simulink model "inner_tanks_init"  (R2020a)
settings: Solver=FixedStepAuto  StartTime=0.0  StopTime=inf  FixedStep=1  RelTol=1e-3
libraries: modbusMatLib x12, simulink x4, realtime_pacer_lib x1
(part 1 of 2)
settings Model: Creator=pppc  LastModifiedBy=Casper and Adis
settings DebuggingCC: InheritedTsInSrcMsg=none
settings SFSimCC: CustomCodeUndefinedFunction=UseInterfaceOnly

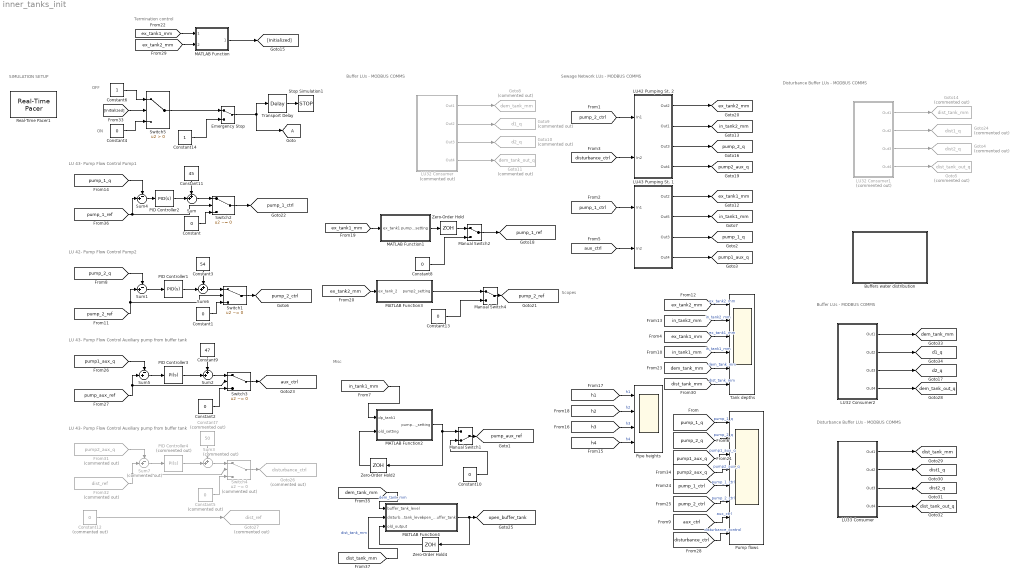
== system inner_tanks_init ==
  note: Buffer LUs - MODBUS COMMS
  note: LU 43- Pump Flow Control Auxiliary pump from buffer tank
  note: OFF
  note: SIMULATION SETUP
  note: Sewage Network LUs - MODBUS COMMS
  note: LU 43- Pump Flow Control Pump1
  note: LU 42- Pump Flow Control Pump2
  note: ON
  note: Scopes
  note: Disturbance Buffer LUs - MODBUS COMMS
  note: LU 43- Pump Flow Control Auxiliary pump from buffer tank
  note: Termination control
  note: Misc
  note: Disturbance Buffer LUs - MODBUS COMMS
  note: Buffer LUs - MODBUS COMMS
  Buffers water distribution : Subsystem
  Constant{,1..2,4,8,10,13} (7 alike) : Constant  Value=0
  Constant11 : Constant  Value=45
  Constant12 : Constant  Commented=on  Value=0
  Constant14 : Constant
  Constant3 : Constant  Value=54
  Constant5 : Constant  Commented=on  Value=0
  Constant6 : Constant
  Constant7 : Constant  Commented=on  Value=50
  Constant9 : Constant  Value=47
  Emergency Stop : ManualSwitch
  From31 : From  Commented=on  GotoTag=pump2_aux_q  TagVisibility=global
  From32 : From  Commented=on  GotoTag=dist_ref  TagVisibility=global
  Goto10 : Goto  Commented=on  GotoTag=d2_q  TagVisibility=global
  Goto11 : Goto  Commented=on  GotoTag=dem_tank_out_q  TagVisibility=global
  Goto14 : Goto  Commented=on  GotoTag=dist_tank_mm  TagVisibility=global
  Goto24 : Goto  Commented=on  GotoTag=dist1_q  TagVisibility=global
  Goto26 : Goto  Commented=on  GotoTag=disturbance_ctrl  TagVisibility=global
  Goto27 : Goto  Commented=on  GotoTag=dist_ref  TagVisibility=global
  Goto4 : Goto  Commented=on  GotoTag=dist2_q  TagVisibility=global
  Goto5 : Goto  Commented=on  GotoTag=dist_tank_out_q  TagVisibility=global
  Goto8 : Goto  Commented=on  GotoTag=dem_tank_mm  TagVisibility=global
  Goto9 : Goto  Commented=on  GotoTag=d1_q  TagVisibility=global
  LU32 Consumer : Subsystem  Commented=on
  LU32 Consumer1 : Subsystem  Commented=on
  LU32 Consumer2 : Subsystem
  LU33 Consumer : Subsystem
  LU42 Pumping St. 2 : Subsystem
  LU43 Pumping St. 1 : Subsystem
  MATLAB Function : MATLAB Function  TreatAsAtomicUnit=on
  MATLAB Function1 : MATLAB Function  TreatAsAtomicUnit=on
  MATLAB Function2 : MATLAB Function  TreatAsAtomicUnit=on
  MATLAB Function3 : MATLAB Function  TreatAsAtomicUnit=on
  MATLAB Function4 : MATLAB Function  TreatAsAtomicUnit=on
  Manual Switch1 : ManualSwitch  CurrentSetting=0
  Manual Switch2 : ManualSwitch
  Manual Switch4 : ManualSwitch
  PID Controller1 : simulink/Continuous/PID Controller  Controller=PID  Form=Parallel  TimeDomain=Continuous-time  UseExternalTs=off  SampleTime=1  IntegratorMethod=Forward Euler  FilterMethod=Forward Euler  ControllerParametersSource=internal  P=0.145  I=0.61  D=0  UseFilter=on  N=100  TunerSelectOption=Transfer Function Based (PID Tuner App)  InitialConditionSource=internal  InitialConditionForIntegrator=0  InitialConditionForFilter=0  DifferentiatorICPrevScaledInput=0  ExternalReset=none  TrackingMode=off  Kt=1  LimitOutput=on  UpperSaturationLimit=46  LowerSaturationLimit=0  LinearizeAsGain=off  AntiWindupMode=clamping  Kb=1  POutMin=[]  POutMax=[]  IOutMin=[]  IOutMax=[]  DOutMin=[]  DOutMax=[]  NOutMin=[]  NOutMax=[]  SumOutMin=[]  SumOutMax=[]  SaturationOutMin=[]  SaturationOutMax=[]  PParamMin=[]  PParamMax=[]  IParamMin=[]  IParamMax=[]  DParamMin=[]  DParamMax=[]  NParamMin=[]  NParamMax=[]  KbParamMin=[]  KbParamMax=[]  KtParamMin=[]  KtParamMax=[]  KbOutMin=[]  KbOutMax=[]  KtOutMin=[]  KtOutMax=[]  IntegratorOutMin=[]  IntegratorOutMax=[]  FilterOutMin=[]  FilterOutMax=[]  SumI1OutMin=[]  SumI1OutMax=[]  SumI2OutMin=[]  SumI2OutMax=[]  SumI3OutMin=[]  SumI3OutMax=[]  SumI4OutMin=[]  SumI4OutMax=[]  SumDOutMin=[]  SumDOutMax=[]  DifferentiatorOutMin=[]  DifferentiatorOutMax=[]  FilterDiffOutCoefMin=[]  FilterDiffOutCoefMax=[]  ReciprocalOutMin=[]  ReciprocalOutMax=[]  SumDenOutMin=[]  SumDenOutMax=[]  SumNumOutMin=[]  SumNumOutMax=[]  DivideOutMin=[]  DivideOutMax=[]  UdiffTsProdOutMin=[]  UdiffTsProdOutMax=[]  NTsProdOutMin=[]  NTsProdOutMax=[]  UintegralTsProdOutMin=[]  UintegralTsProdOutMax=[]  UngainTsProdOutMin=[]  UngainTsProdOutMax=[]  IntegratorContinuousStateAttributes=''  IntegratorStateMustResolveToSignalObject=off  IntegratorRTWStateStorageClass=Auto  FilterContinuousStateAttributes=''  FilterStateMustResolveToSignalObject=off  FilterRTWStateStorageClass=Auto  ParallelPVariant=InternalParameters  IdealPVariant=Disabled  IVariant=InternalParameters  DVariant=InternalParameters  IntegratorVariant=Continuous  SatVariant=Enabled  AWVariant=ContClampingParallel  PCopyVariant=Disabled  TRVariant=Disabled  FdbkBlocksVariant=Forward  IdealPFdbkVariant=Disabled  SatFdbkVariant=Disabled  DerivativeFilterVariant=ContFilter  NVariant=InternalParameters  NCopyVariant=Disabled  FilterICVariant=InternalICsFilter  IntegratorICVariant=InternalICs  ExternalResetVariant=Disabled  TRSumVariant=Passthrough  SumFdbkVariant=Disabled  SumVariant=Sum_PID  TsampFilterVariant=InternalTs  TsampNgainVariant=Passthrough  TsampIntegralVariant=Passthrough
  PID Controller2 : simulink/Continuous/PID Controller  Controller=PID  Form=Parallel  TimeDomain=Continuous-time  UseExternalTs=off  SampleTime=1  IntegratorMethod=Forward Euler  FilterMethod=Forward Euler  ControllerParametersSource=internal  P=0.1  I=0.3  D=0  UseFilter=on  N=100  TunerSelectOption=Transfer Function Based (PID Tuner App)  InitialConditionSource=internal  InitialConditionForIntegrator=0  InitialConditionForFilter=0  DifferentiatorICPrevScaledInput=0  ExternalReset=none  TrackingMode=off  Kt=1  LimitOutput=on  UpperSaturationLimit=49  LowerSaturationLimit=0  LinearizeAsGain=off  AntiWindupMode=clamping  Kb=1  POutMin=[]  POutMax=[]  IOutMin=[]  IOutMax=[]  DOutMin=[]  DOutMax=[]  NOutMin=[]  NOutMax=[]  SumOutMin=[]  SumOutMax=[]  SaturationOutMin=[]  SaturationOutMax=[]  PParamMin=[]  PParamMax=[]  IParamMin=[]  IParamMax=[]  DParamMin=[]  DParamMax=[]  NParamMin=[]  NParamMax=[]  KbParamMin=[]  KbParamMax=[]  KtParamMin=[]  KtParamMax=[]  KbOutMin=[]  KbOutMax=[]  KtOutMin=[]  KtOutMax=[]  IntegratorOutMin=[]  IntegratorOutMax=[]  FilterOutMin=[]  FilterOutMax=[]  SumI1OutMin=[]  SumI1OutMax=[]  SumI2OutMin=[]  SumI2OutMax=[]  SumI3OutMin=[]  SumI3OutMax=[]  SumI4OutMin=[]  SumI4OutMax=[]  SumDOutMin=[]  SumDOutMax=[]  DifferentiatorOutMin=[]  DifferentiatorOutMax=[]  FilterDiffOutCoefMin=[]  FilterDiffOutCoefMax=[]  ReciprocalOutMin=[]  ReciprocalOutMax=[]  SumDenOutMin=[]  SumDenOutMax=[]  SumNumOutMin=[]  SumNumOutMax=[]  DivideOutMin=[]  DivideOutMax=[]  UdiffTsProdOutMin=[]  UdiffTsProdOutMax=[]  NTsProdOutMin=[]  NTsProdOutMax=[]  UintegralTsProdOutMin=[]  UintegralTsProdOutMax=[]  UngainTsProdOutMin=[]  UngainTsProdOutMax=[]  IntegratorContinuousStateAttributes=''  IntegratorStateMustResolveToSignalObject=off  IntegratorRTWStateStorageClass=Auto  FilterContinuousStateAttributes=''  FilterStateMustResolveToSignalObject=off  FilterRTWStateStorageClass=Auto  ParallelPVariant=InternalParameters  IdealPVariant=Disabled  IVariant=InternalParameters  DVariant=InternalParameters  IntegratorVariant=Continuous  SatVariant=Enabled  AWVariant=ContClampingParallel  PCopyVariant=Disabled  TRVariant=Disabled  FdbkBlocksVariant=Forward  IdealPFdbkVariant=Disabled  SatFdbkVariant=Disabled  DerivativeFilterVariant=ContFilter  NVariant=InternalParameters  NCopyVariant=Disabled  FilterICVariant=InternalICsFilter  IntegratorICVariant=InternalICs  ExternalResetVariant=Disabled  TRSumVariant=Passthrough  SumFdbkVariant=Disabled  SumVariant=Sum_PID  TsampFilterVariant=InternalTs  TsampNgainVariant=Passthrough  TsampIntegralVariant=Passthrough
  PID Controller3 : simulink/Continuous/PID Controller  Controller=PI  Form=Parallel  TimeDomain=Continuous-time  UseExternalTs=off  SampleTime=1  IntegratorMethod=Forward Euler  FilterMethod=Forward Euler  ControllerParametersSource=internal  P=0.15  I=0.45  D=0  UseFilter=on  N=100  TunerSelectOption=Transfer Function Based (PID Tuner App)  InitialConditionSource=internal  InitialConditionForIntegrator=0  InitialConditionForFilter=0  DifferentiatorICPrevScaledInput=0  ExternalReset=none  TrackingMode=off  Kt=1  LimitOutput=on  UpperSaturationLimit=53  LowerSaturationLimit=0  LinearizeAsGain=off  AntiWindupMode=clamping  Kb=1  POutMin=[]  POutMax=[]  IOutMin=[]  IOutMax=[]  DOutMin=[]  DOutMax=[]  NOutMin=[]  NOutMax=[]  SumOutMin=[]  SumOutMax=[]  SaturationOutMin=[]  SaturationOutMax=[]  PParamMin=[]  PParamMax=[]  IParamMin=[]  IParamMax=[]  DParamMin=[]  DParamMax=[]  NParamMin=[]  NParamMax=[]  KbParamMin=[]  KbParamMax=[]  KtParamMin=[]  KtParamMax=[]  KbOutMin=[]  KbOutMax=[]  KtOutMin=[]  KtOutMax=[]  IntegratorOutMin=[]  IntegratorOutMax=[]  FilterOutMin=[]  FilterOutMax=[]  SumI1OutMin=[]  SumI1OutMax=[]  SumI2OutMin=[]  SumI2OutMax=[]  SumI3OutMin=[]  SumI3OutMax=[]  SumI4OutMin=[]  SumI4OutMax=[]  SumDOutMin=[]  SumDOutMax=[]  DifferentiatorOutMin=[]  DifferentiatorOutMax=[]  FilterDiffOutCoefMin=[]  FilterDiffOutCoefMax=[]  ReciprocalOutMin=[]  ReciprocalOutMax=[]  SumDenOutMin=[]  SumDenOutMax=[]  SumNumOutMin=[]  SumNumOutMax=[]  DivideOutMin=[]  DivideOutMax=[]  UdiffTsProdOutMin=[]  UdiffTsProdOutMax=[]  NTsProdOutMin=[]  NTsProdOutMax=[]  UintegralTsProdOutMin=[]  UintegralTsProdOutMax=[]  UngainTsProdOutMin=[]  UngainTsProdOutMax=[]  IntegratorContinuousStateAttributes=''  IntegratorStateMustResolveToSignalObject=off  IntegratorRTWStateStorageClass=Auto  FilterContinuousStateAttributes=''  FilterStateMustResolveToSignalObject=off  FilterRTWStateStorageClass=Auto  ParallelPVariant=InternalParameters  IdealPVariant=Disabled  IVariant=InternalParameters  DVariant=Disabled  IntegratorVariant=Continuous  SatVariant=Enabled  AWVariant=ContClampingParallel  PCopyVariant=Disabled  TRVariant=Disabled  FdbkBlocksVariant=Forward  IdealPFdbkVariant=Disabled  SatFdbkVariant=Disabled  DerivativeFilterVariant=Disabled  NVariant=Disabled  NCopyVariant=Disabled_SignalSpec  FilterICVariant=Disabled  IntegratorICVariant=InternalICs  ExternalResetVariant=Disabled  TRSumVariant=Passthrough  SumFdbkVariant=Disabled  SumVariant=Sum_PI  TsampFilterVariant=InternalTs  TsampNgainVariant=Passthrough  TsampIntegralVariant=Passthrough
  PID Controller4 : simulink/Continuous/PID Controller  Commented=on  Controller=PI  Form=Parallel  TimeDomain=Continuous-time  UseExternalTs=off  SampleTime=1  IntegratorMethod=Forward Euler  FilterMethod=Forward Euler  ControllerParametersSource=internal  P=0.1  I=0.4  D=0  UseFilter=on  N=100  TunerSelectOption=Transfer Function Based (PID Tuner App)  InitialConditionSource=internal  InitialConditionForIntegrator=0  InitialConditionForFilter=0  DifferentiatorICPrevScaledInput=0  ExternalReset=none  TrackingMode=off  Kt=1  LimitOutput=on  UpperSaturationLimit=53  LowerSaturationLimit=0  LinearizeAsGain=off  AntiWindupMode=clamping  Kb=1  POutMin=[]  POutMax=[]  IOutMin=[]  IOutMax=[]  DOutMin=[]  DOutMax=[]  NOutMin=[]  NOutMax=[]  SumOutMin=[]  SumOutMax=[]  SaturationOutMin=[]  SaturationOutMax=[]  PParamMin=[]  PParamMax=[]  IParamMin=[]  IParamMax=[]  DParamMin=[]  DParamMax=[]  NParamMin=[]  NParamMax=[]  KbParamMin=[]  KbParamMax=[]  KtParamMin=[]  KtParamMax=[]  KbOutMin=[]  KbOutMax=[]  KtOutMin=[]  KtOutMax=[]  IntegratorOutMin=[]  IntegratorOutMax=[]  FilterOutMin=[]  FilterOutMax=[]  SumI1OutMin=[]  SumI1OutMax=[]  SumI2OutMin=[]  SumI2OutMax=[]  SumI3OutMin=[]  SumI3OutMax=[]  SumI4OutMin=[]  SumI4OutMax=[]  SumDOutMin=[]  SumDOutMax=[]  DifferentiatorOutMin=[]  DifferentiatorOutMax=[]  FilterDiffOutCoefMin=[]  FilterDiffOutCoefMax=[]  ReciprocalOutMin=[]  ReciprocalOutMax=[]  SumDenOutMin=[]  SumDenOutMax=[]  SumNumOutMin=[]  SumNumOutMax=[]  DivideOutMin=[]  DivideOutMax=[]  UdiffTsProdOutMin=[]  UdiffTsProdOutMax=[]  NTsProdOutMin=[]  NTsProdOutMax=[]  UintegralTsProdOutMin=[]  UintegralTsProdOutMax=[]  UngainTsProdOutMin=[]  UngainTsProdOutMax=[]  IntegratorContinuousStateAttributes=''  IntegratorStateMustResolveToSignalObject=off  IntegratorRTWStateStorageClass=Auto  FilterContinuousStateAttributes=''  FilterStateMustResolveToSignalObject=off  FilterRTWStateStorageClass=Auto  ParallelPVariant=InternalParameters  IdealPVariant=Disabled  IVariant=InternalParameters  DVariant=Disabled  IntegratorVariant=Continuous  SatVariant=Enabled  AWVariant=ContClampingParallel  PCopyVariant=Disabled  TRVariant=Disabled  FdbkBlocksVariant=Forward  IdealPFdbkVariant=Disabled  SatFdbkVariant=Disabled  DerivativeFilterVariant=Disabled  NVariant=Disabled  NCopyVariant=Disabled_SignalSpec  FilterICVariant=Disabled  IntegratorICVariant=InternalICs  ExternalResetVariant=Disabled  TRSumVariant=Passthrough  SumFdbkVariant=Disabled  SumVariant=Sum_PI  TsampFilterVariant=InternalTs  TsampNgainVariant=Passthrough  TsampIntegralVariant=Passthrough
  Pipe heights : Scope  NumInputPorts=4
  Pump flows : Scope  NumInputPorts=8
  Real-Time Pacer1 : realtime_pacer_lib/Real-Time Pacer  simTimePerRealTime=2
  Stop Simulation1 : Stop
  Sum : Sum  Inputs=++|
  Sum1 : Sum  Inputs=-+|
  Sum2 : Sum  Inputs=++|
  Sum3 : Sum  Commented=on  Inputs=++|
  Sum4 : Sum  Inputs=-+|
  Sum5 : Sum  Inputs=-+|
  Sum6 : Sum  Inputs=++|
  Sum7 : Sum  Commented=on  Inputs=-+|
  Switch1 : Switch  Criteria=u2 ~= 0
  Switch2 : Switch  Criteria=u2 ~= 0
  Switch3 : Switch  Criteria=u2 ~= 0
  Switch4 : Switch  Commented=on  Criteria=u2 ~= 0
  Switch5 : Switch  Criteria=u2 > Threshold
  Tank depths : Scope  NumInputPorts=6
  Transport Delay : TransportDelay  DelayTime=2
  Zero-Order Hold : ZeroOrderHold  SampleTime=60
  Zero-Order Hold2 : ZeroOrderHold  SampleTime=2
  Zero-Order Hold4 : ZeroOrderHold  SampleTime=2
  tag scope: A=global, aux_ctrl=global, d1_q=global, d2_q=global, dem_tank_mm=global, dem_tank_out_q=global, dist1_q=global, dist2_q=global, dist_tank_mm=global, dist_tank_out_q=global, ex_tank1_mm=global, ex_tank2_mm=global, in_tank1_mm=global, in_tank2_mm=global, open_buffer_tank=global, pump1_aux_q=global, pump2_aux_q=global, pump_1_ctrl=global, pump_1_q=global, pump_1_ref=global, pump_2_ctrl=global, pump_2_q=global, pump_2_ref=global, pump_aux_ref=global
  wires:
  [pump_1_q] -> Sum4/1
  [pump_aux_ref] -> Sum5/2, Switch3/2
  [disturbance_ctrl] -> LU42 Pumping St. 2/2(In2)
  [pump_2_ref] -> Switch1/2, Sum1/2
  [in_tank2_mm] -> Tank depths/2  "in_tank2_mm"
  [pump_2_q] -> Pump flows/2  "pump_2_q"
  Switch1/1 -> [pump_2_ctrl]
  Sum6/1 -> Switch1/1
  PID Controller2/1 -> Sum/2
  PID Controller1/1 -> Sum6/2
  Switch3/1 -> [aux_ctrl]
  [pump_2_q] -> Sum1/1
  Sum2/1 -> Switch3/1
  LU42 Pumping St. 2/3(Out3) -> [pump_2_q]
  Constant9/1 -> Sum2/1
  LU32 Consumer/4(Out4) -> Goto11/1
  Constant2/1 -> Switch3/3
  PID Controller3/1 -> Sum2/2
  [h4] -> Pipe heights/4  "h4"
  Constant11/1 -> Sum/1
  [pump_1_ref] -> Sum4/2, Switch2/2
  [pump_1_ctrl] -> LU43 Pumping St. 1/1(In1)
  Constant3/1 -> Sum6/1
  LU43 Pumping St. 1/2(Out5) -> [in_tank1_mm]
  Sum/1 -> Switch2/1
  Transport Delay/1 -> Stop Simulation1/1
  Constant/1 -> Switch2/3
  LU43 Pumping St. 1/1(Out2) -> [ex_tank1_mm]
  [in_tank1_mm] -> Tank depths/4  "in_tank1_mm"
  [ex_tank1_mm] -> Tank depths/3  "ex_tank1_mm"
  [pump1_aux_q] -> Sum5/1
  [dem_tank_mm] -> Tank depths/5  "dem_tank_mm"
  Sum5/1 -> PID Controller3/1
  [pump_2_ctrl] -> LU42 Pumping St. 2/1(In1)
  LU42 Pumping St. 2/4(Out4) -> [pump2_aux_q]
  LU32 Consumer/3(Out3) -> Goto10/1
  LU32 Consumer/1(Out1) -> Goto8/1
  LU42 Pumping St. 2/1(Out2) -> [ex_tank2_mm]
  [ex_tank1_mm] -> MATLAB Function1/1(ex_tank1)
  Sum1/1 -> PID Controller1/1
  [ex_tank2_mm] -> Tank depths/1  "ex_tank2_mm"
  Switch2/1 -> [pump_1_ctrl]
  [h2] -> Pipe heights/2  "h2"
  [h3] -> Pipe heights/3  "h3"
  LU43 Pumping St. 1/3(Out3) -> [pump_1_q]
  Sum4/1 -> PID Controller2/1
  LU43 Pumping St. 1/4(Out4) -> [pump1_aux_q]
  [aux_ctrl] -> LU43 Pumping St. 1/2(In2)
  LU42 Pumping St. 2/2(Out1) -> [in_tank2_mm]
  LU32 Consumer/2(Out2) -> Goto9/1
  MATLAB Function1/1(pump1_setting) -> Zero-Order Hold/1
  Constant1/1 -> Switch1/3
  [in_tank1_mm] -> MATLAB Function2/1(dp_tank1)
  MATLAB Function2/1(pump_aux_setting) -> Manual Switch1/1, Zero-Order Hold2/1
  Zero-Order Hold2/1 -> MATLAB Function2/2(old_setting)
  [pump1_aux_q] -> Pump flows/3  "pump1_aux_q"
  [pump_1_q] -> Pump flows/1  "pump_1_q"
  LU32 Consumer1/2(Out2) -> Goto24/1
  LU32 Consumer1/3(Out3) -> Goto4/1
  LU32 Consumer1/4(Out4) -> Goto5/1
  LU32 Consumer1/1(Out1) -> Goto14/1
  [dist_tank_mm] -> Tank depths/6  "dist_tank_mm"
  From31/1 -> Sum7/1
  Constant7/1 -> Sum3/1
  Switch4/1 -> Goto26/1
  PID Controller4/1 -> Sum3/2
  From32/1 -> Sum7/2, Switch4/2
  Sum3/1 -> Switch4/1
  Sum7/1 -> PID Controller4/1
  Constant5/1 -> Switch4/3
  [pump_1_ctrl] -> Pump flows/5  "pump_1_ctrl"
  [pump_2_ctrl] -> Pump flows/6  "pump_2_ctrl"
  [aux_ctrl] -> Pump flows/7  "aux_ctrl"
  [disturbance_ctrl] -> Pump flows/8  "disturbance_control"
  [pump2_aux_q] -> Pump flows/4  "pump2_aux_q"
  [dem_tank_mm] -> MATLAB Function4/1(buffer_tank_level)  "dem_tank_mm"
  [dist_tank_mm] -> MATLAB Function4/2(disturbance_tank_level)  "dist_tank_mm"
  MATLAB Function4/1(open_buffer_tank) -> Zero-Order Hold4/1, [open_buffer_tank]
  Zero-Order Hold4/1 -> MATLAB Function4/3(old_output)
  [h1] -> Pipe heights/1  "h1"
  Constant12/1 -> Goto27/1
  Emergency Stop/1 -> Transport Delay/1, [A]
  Manual Switch1/1 -> [pump_aux_ref]
  Constant10/1 -> Manual Switch1/2
  Zero-Order Hold/1 -> Manual Switch2/1
  Manual Switch2/1 -> [pump_1_ref]
  Constant8/1 -> Manual Switch2/2
  [ex_tank2_mm] -> MATLAB Function3/1(ex_tank_2)
  MATLAB Function3/1(pump2_setting) -> Manual Switch4/1
  Manual Switch4/1 -> [pump_2_ref]
  Constant13/1 -> Manual Switch4/2
  [ex_tank1_mm] -> MATLAB Function/1(ex_tank1)
  [ex_tank2_mm] -> MATLAB Function/2(ex_tank2)
  MATLAB Function/1(initialized) -> [Initialized]
  Constant6/1 -> Switch5/1
  Constant4/1 -> Switch5/3
  [Initialized] -> Switch5/2
  Constant14/1 -> Emergency Stop/2
  Switch5/1 -> Emergency Stop/1
  LU32 Consumer2/4(Out4) -> [dem_tank_out_q]
  LU33 Consumer/2(Out2) -> [dist1_q]
  LU32 Consumer2/3(Out3) -> [d2_q]
  LU33 Consumer/4(Out4) -> [dist_tank_out_q]
  LU33 Consumer/1(Out1) -> [dist_tank_mm]
  LU32 Consumer2/1(Out1) -> [dem_tank_mm]
  LU33 Consumer/3(Out3) -> [dist2_q]
  LU32 Consumer2/2(Out2) -> [d1_q]

== system inner_tanks_init/Buffers water distribution ==
  Constant : Constant
  Debug purposes : Constant  Value=0
  Delay : Delay  SampleTime=1
  MATLAB Function4 : MATLAB Function  TreatAsAtomicUnit=on
  Manual Switch : ManualSwitch  CurrentSetting=0
  Manual Switch1 : ManualSwitch
  tag scope: tank_select=global
  wires:
  [dem_tank_mm] -> MATLAB Function4/1(buffer_tank_level)  "dem_tank_mm"
  MATLAB Function4/1(tank_select) -> Delay/1, Manual Switch/2
  [dist_tank_mm] -> MATLAB Function4/2(disturbance_tank_level)  "dist_tank_mm"
  Manual Switch/1 -> [tank_select]
  Manual Switch1/1 -> Manual Switch/1
  Constant/1 -> Manual Switch1/1
  Debug purposes/1 -> Manual Switch1/2
  Delay/1 -> MATLAB Function4/3(old_output)

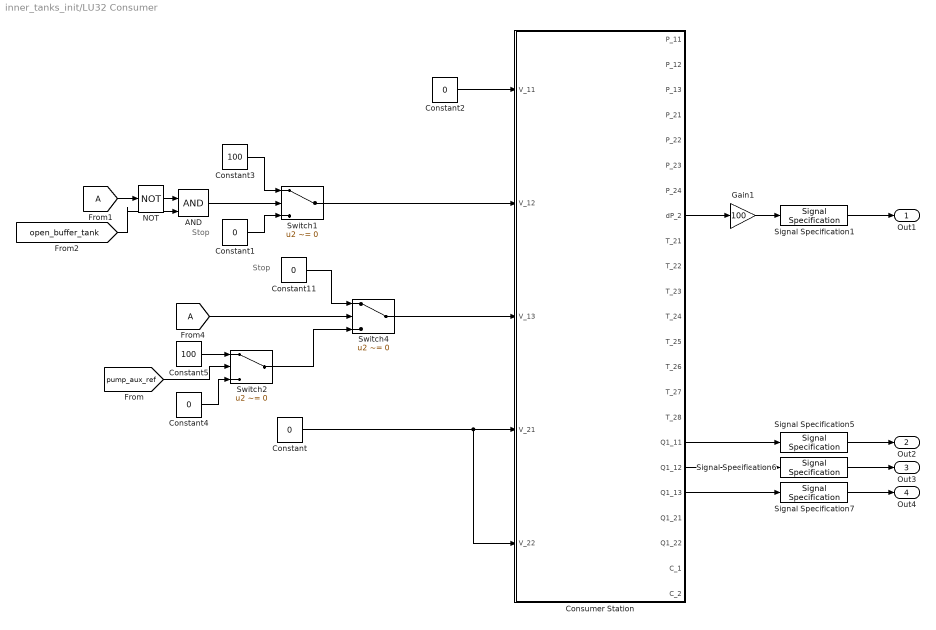
== system inner_tanks_init/LU32 Consumer ==
  note: Stop
  note: Stop
  AND : Logic  IconShape=distinctive  AllPortsSameDT=off  OutDataTypeStr=boolean
  Constant{,1..2,4,11} (5 alike) : Constant  Value=0
  Constant3 : Constant  Value=100
  Constant5 : Constant  Value=100
  Consumer Station : Subsystem
  Gain1 : Gain  Gain=100
  NOT : Logic  Operator=NOT  IconShape=distinctive  AllPortsSameDT=off  OutDataTypeStr=boolean
  Signal Specification1 : SignalSpecification  Unit=mm
  Signal Specification5 : SignalSpecification  Unit=l/min
  Signal Specification6 : SignalSpecification  Unit=l/min
  Signal Specification7 : SignalSpecification  Unit=l/min
  Switch1 : Switch  Criteria=u2 ~= 0
  Switch2 : Switch  Criteria=u2 ~= 0
  Switch4 : Switch  Criteria=u2 ~= 0
  Out1 : Outport  VectorParamsAs1DForOutWhenUnconnected=off
  Out2 : Outport  Port=2  VectorParamsAs1DForOutWhenUnconnected=off
  Out3 : Outport  Port=3  VectorParamsAs1DForOutWhenUnconnected=off
  Out4 : Outport  Port=4  VectorParamsAs1DForOutWhenUnconnected=off
  wires:
  Consumer Station/8(dP_2) -> Gain1/1
  Switch4/1 -> Consumer Station/3(V_13)
  Consumer Station/19(Q1_13) -> Signal Specification7/1
  Consumer Station/17(Q1_11) -> Signal Specification5/1
  Consumer Station/18(Q1_12) -> Signal Specification6/1
  Gain1/1 -> Signal Specification1/1
  [A] -> Switch4/2
  Signal Specification7/1 -> Out4/1
  Constant11/1 -> Switch4/1
  Signal Specification5/1 -> Out2/1
  Constant/1 -> Consumer Station/5(V_22), Consumer Station/4(V_21)
  Signal Specification6/1 -> Out3/1
  Signal Specification1/1 -> Out1/1
  Switch1/1 -> Consumer Station/2(V_12)
  Constant2/1 -> Consumer Station/1(V_11)
  [pump_aux_ref] -> Switch2/2
  Switch2/1 -> Switch4/3
  Constant5/1 -> Switch2/1
  Constant4/1 -> Switch2/3
  [A] -> NOT/1
  NOT/1 -> AND/1
  AND/1 -> Switch1/2
  Constant1/1 -> Switch1/3
  Constant3/1 -> Switch1/1
  [open_buffer_tank] -> AND/2

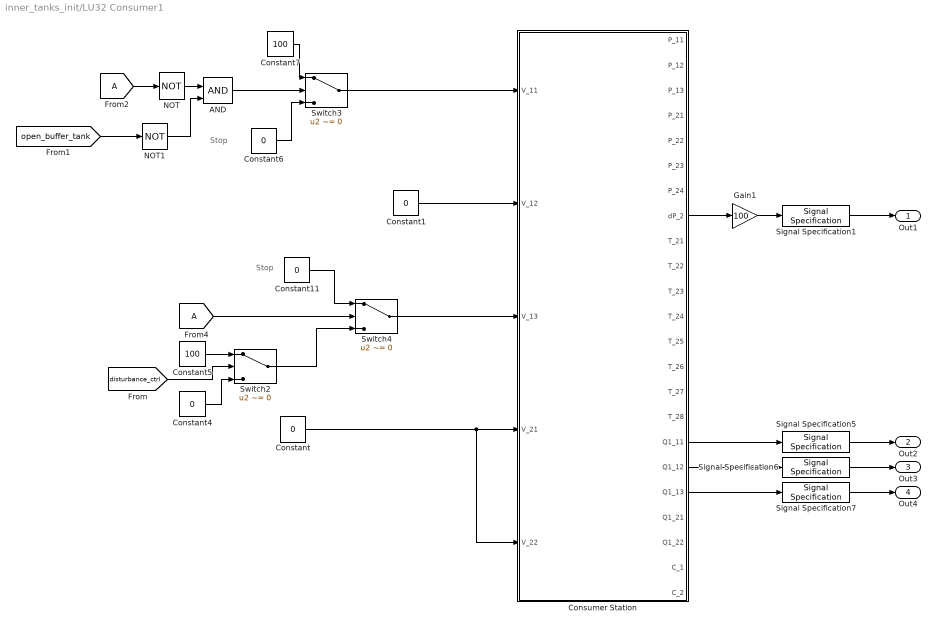
== system inner_tanks_init/LU32 Consumer1 ==
  note: Stop
  note: Stop
  AND : Logic  IconShape=distinctive  AllPortsSameDT=off  OutDataTypeStr=boolean
  Constant{,1,4,6,11} (5 alike) : Constant  Value=0
  Constant5 : Constant  Value=100
  Constant7 : Constant  Value=100
  Consumer Station : Subsystem
  Gain1 : Gain  Gain=100
  NOT : Logic  Operator=NOT  IconShape=distinctive  AllPortsSameDT=off  OutDataTypeStr=boolean
  NOT1 : Logic  Operator=NOT  IconShape=distinctive  AllPortsSameDT=off  OutDataTypeStr=boolean
  Signal Specification1 : SignalSpecification  Unit=mm
  Signal Specification5 : SignalSpecification  Unit=l/min
  Signal Specification6 : SignalSpecification  Unit=l/min
  Signal Specification7 : SignalSpecification  Unit=l/min
  Switch2 : Switch  Criteria=u2 ~= 0
  Switch3 : Switch  Criteria=u2 ~= 0
  Switch4 : Switch  Criteria=u2 ~= 0
  Out1 : Outport  VectorParamsAs1DForOutWhenUnconnected=off
  Out2 : Outport  Port=2  VectorParamsAs1DForOutWhenUnconnected=off
  Out3 : Outport  Port=3  VectorParamsAs1DForOutWhenUnconnected=off
  Out4 : Outport  Port=4  VectorParamsAs1DForOutWhenUnconnected=off
  wires:
  Consumer Station/8(dP_2) -> Gain1/1
  Switch4/1 -> Consumer Station/3(V_13)
  Consumer Station/19(Q1_13) -> Signal Specification7/1
  Consumer Station/17(Q1_11) -> Signal Specification5/1
  Consumer Station/18(Q1_12) -> Signal Specification6/1
  Gain1/1 -> Signal Specification1/1
  [A] -> Switch4/2
  Signal Specification7/1 -> Out4/1
  Constant11/1 -> Switch4/1
  Signal Specification5/1 -> Out2/1
  Constant/1 -> Consumer Station/5(V_22), Consumer Station/4(V_21)
  Signal Specification6/1 -> Out3/1
  Signal Specification1/1 -> Out1/1
  Switch3/1 -> Consumer Station/1(V_11)
  [disturbance_ctrl] -> Switch2/2
  Switch2/1 -> Switch4/3
  Constant5/1 -> Switch2/1
  Constant4/1 -> Switch2/3
  Constant1/1 -> Consumer Station/2(V_12)
  [A] -> NOT/1
  Constant6/1 -> Switch3/3
  Constant7/1 -> Switch3/1
  AND/1 -> Switch3/2
  NOT/1 -> AND/1
  [open_buffer_tank] -> NOT1/1
  NOT1/1 -> AND/2

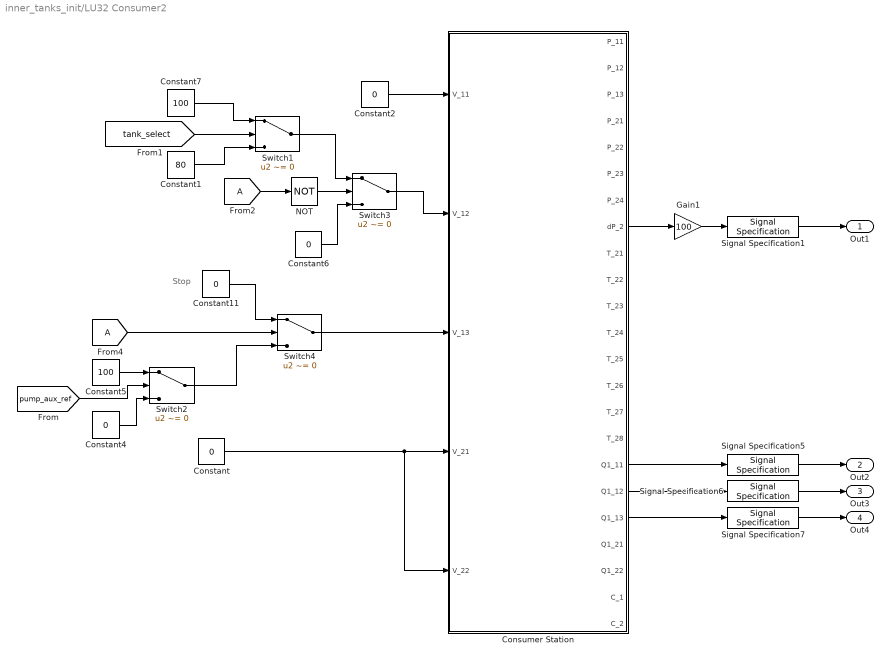
== system inner_tanks_init/LU32 Consumer2 ==
  note: Stop
  Constant{,2,4,6,11} (5 alike) : Constant  Value=0
  Constant1 : Constant  Value=80
  Constant5 : Constant  Value=100
  Constant7 : Constant  Value=100
  Consumer Station : Subsystem
  Gain1 : Gain  Gain=100
  NOT : Logic  Operator=NOT  IconShape=distinctive  AllPortsSameDT=off  OutDataTypeStr=boolean
  Signal Specification1 : SignalSpecification  Unit=mm
  Signal Specification5 : SignalSpecification  Unit=l/min
  Signal Specification6 : SignalSpecification  Unit=l/min
  Signal Specification7 : SignalSpecification  Unit=l/min
  Switch{1..4} (4 alike) : Switch  Criteria=u2 ~= 0
  Out1 : Outport  VectorParamsAs1DForOutWhenUnconnected=off
  Out2 : Outport  Port=2  VectorParamsAs1DForOutWhenUnconnected=off
  Out3 : Outport  Port=3  VectorParamsAs1DForOutWhenUnconnected=off
  Out4 : Outport  Port=4  VectorParamsAs1DForOutWhenUnconnected=off
  wires:
  Consumer Station/8(dP_2) -> Gain1/1
  Switch4/1 -> Consumer Station/3(V_13)
  Consumer Station/19(Q1_13) -> Signal Specification7/1
  Consumer Station/17(Q1_11) -> Signal Specification5/1
  Consumer Station/18(Q1_12) -> Signal Specification6/1
  Gain1/1 -> Signal Specification1/1
  [A] -> Switch4/2
  Signal Specification7/1 -> Out4/1
  Constant11/1 -> Switch4/1
  Signal Specification5/1 -> Out2/1
  Constant/1 -> Consumer Station/5(V_22), Consumer Station/4(V_21)
  Signal Specification6/1 -> Out3/1
  Signal Specification1/1 -> Out1/1
  Constant2/1 -> Consumer Station/1(V_11)
  [pump_aux_ref] -> Switch2/2
  Switch2/1 -> Switch4/3
  Constant5/1 -> Switch2/1
  Constant4/1 -> Switch2/3
  Constant6/1 -> Switch3/3
  [tank_select] -> Switch1/2
  Constant1/1 -> Switch1/3
  NOT/1 -> Switch3/2
  [A] -> NOT/1
  Switch3/1 -> Consumer Station/2(V_12)
  Switch1/1 -> Switch3/1
  Constant7/1 -> Switch1/1

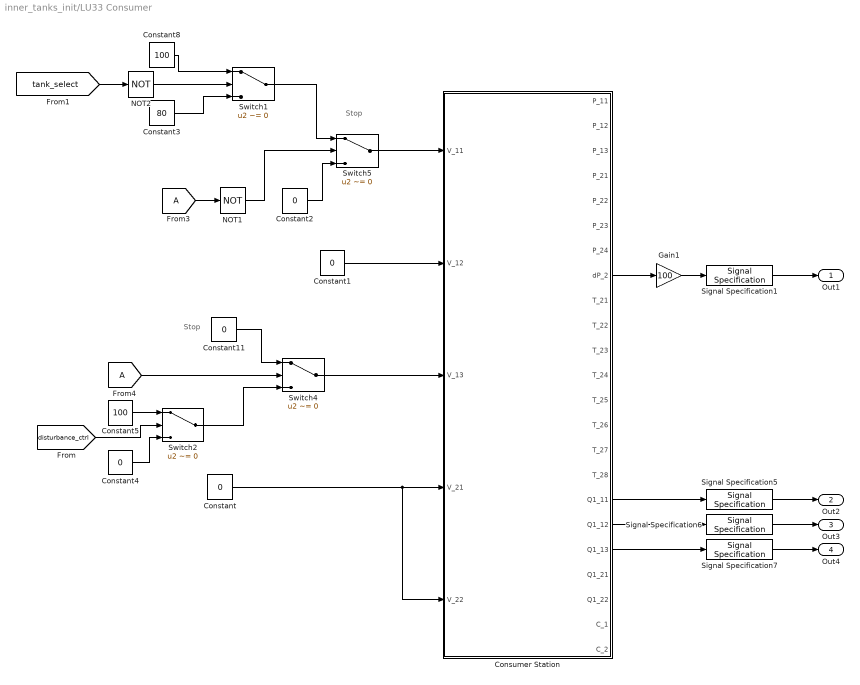
== system inner_tanks_init/LU33 Consumer ==
  note: Stop
  note: Stop
  Constant{,1..2,4,11} (5 alike) : Constant  Value=0
  Constant3 : Constant  Value=80
  Constant5 : Constant  Value=100
  Constant8 : Constant  Value=100
  Consumer Station : Subsystem
  Gain1 : Gain  Gain=100
  NOT1 : Logic  Operator=NOT  IconShape=distinctive  AllPortsSameDT=off  OutDataTypeStr=boolean
  NOT2 : Logic  Operator=NOT  IconShape=distinctive  AllPortsSameDT=off  OutDataTypeStr=boolean
  Signal Specification1 : SignalSpecification  Unit=mm
  Signal Specification5 : SignalSpecification  Unit=l/min
  Signal Specification6 : SignalSpecification  Unit=l/min
  Signal Specification7 : SignalSpecification  Unit=l/min
  Switch{1..2,4..5} (4 alike) : Switch  Criteria=u2 ~= 0
  Out1 : Outport  VectorParamsAs1DForOutWhenUnconnected=off
  Out2 : Outport  Port=2  VectorParamsAs1DForOutWhenUnconnected=off
  Out3 : Outport  Port=3  VectorParamsAs1DForOutWhenUnconnected=off
  Out4 : Outport  Port=4  VectorParamsAs1DForOutWhenUnconnected=off
  wires:
  Consumer Station/8(dP_2) -> Gain1/1
  Switch4/1 -> Consumer Station/3(V_13)
  Consumer Station/19(Q1_13) -> Signal Specification7/1
  Consumer Station/17(Q1_11) -> Signal Specification5/1
  Consumer Station/18(Q1_12) -> Signal Specification6/1
  Gain1/1 -> Signal Specification1/1
  [A] -> Switch4/2
  Signal Specification7/1 -> Out4/1
  Constant11/1 -> Switch4/1
  Signal Specification5/1 -> Out2/1
  Constant/1 -> Consumer Station/5(V_22), Consumer Station/4(V_21)
  Signal Specification6/1 -> Out3/1
  Signal Specification1/1 -> Out1/1
  [disturbance_ctrl] -> Switch2/2
  Switch2/1 -> Switch4/3
  Constant5/1 -> Switch2/1
  Constant4/1 -> Switch2/3
  Constant1/1 -> Consumer Station/2(V_12)
  Switch1/1 -> Switch5/1
  Constant8/1 -> Switch1/1
  NOT1/1 -> Switch5/2
  NOT2/1 -> Switch1/2
  Constant2/1 -> Switch5/3
  [tank_select] -> NOT2/1
  Switch5/1 -> Consumer Station/1(V_11)
  [A] -> NOT1/1
  Constant3/1 -> Switch1/3

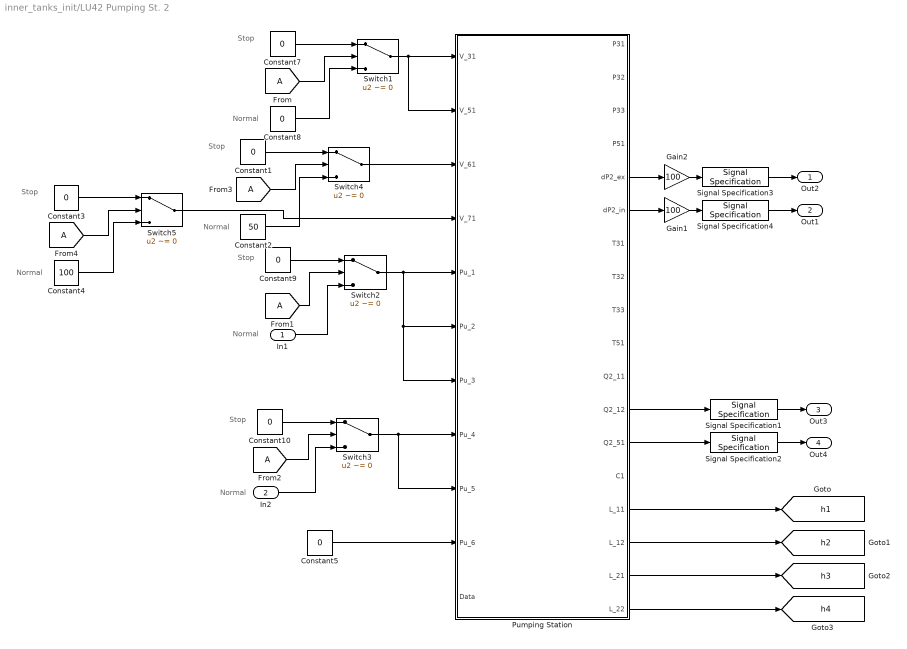
== system inner_tanks_init/LU42 Pumping St. 2 ==
  note: Stop
  note: Stop
  note: Normal
  note: Stop
  note: Normal
  note: Normal
  note: Stop
  note: Normal
  note: Normal
  note: Stop
  In1 : Inport
  In2 : Inport  Port=2
  Constant{1,3,5,7..10} (7 alike) : Constant  Value=0
  Constant2 : Constant  Value=50
  Constant4 : Constant  Value=100
  Gain1 : Gain  Gain=100
  Gain2 : Gain  Gain=100
  Pumping Station : Subsystem
  Signal Specification1 : SignalSpecification  Unit=l/min
  Signal Specification2 : SignalSpecification  Unit=l/min
  Signal Specification3 : SignalSpecification  Unit=mm
  Signal Specification4 : SignalSpecification  Unit=mm
  Switch{1..5} (5 alike) : Switch  Criteria=u2 ~= 0
  Out2 : Outport  VectorParamsAs1DForOutWhenUnconnected=off
  Out1 : Outport  Port=2  VectorParamsAs1DForOutWhenUnconnected=off
  Out3 : Outport  Port=3  VectorParamsAs1DForOutWhenUnconnected=off
  Out4 : Outport  Port=4  VectorParamsAs1DForOutWhenUnconnected=off
  tag scope: h1=global, h2=global, h3=global, h4=global
  wires:
  Switch2/1 -> Pumping Station/7(Pu_3), Pumping Station/6(Pu_2), Pumping Station/5(Pu_1)
  [A] -> Switch1/2
  Constant7/1 -> Switch1/1
  Constant8/1 -> Switch1/3
  Switch3/1 -> Pumping Station/9(Pu_5), Pumping Station/8(Pu_4)
  Constant10/1 -> Switch3/1
  In1/1 -> Switch2/3
  [A] -> Switch2/2
  Constant9/1 -> Switch2/1
  In2/1 -> Switch3/3
  Gain2/1 -> Signal Specification3/1
  Constant5/1 -> Pumping Station/10(Pu_6)
  Signal Specification3/1 -> Out2/1
  [A] -> Switch3/2
  Pumping Station/5(dP2_ex) -> Gain2/1
  Switch1/1 -> Pumping Station/2(V_51), Pumping Station/1(V_31)
  Signal Specification1/1 -> Out3/1
  Signal Specification2/1 -> Out4/1
  Pumping Station/12(Q2_12) -> Signal Specification1/1
  Pumping Station/13(Q2_51) -> Signal Specification2/1
  Pumping Station/6(dP2_in) -> Gain1/1
  Gain1/1 -> Signal Specification4/1
  Signal Specification4/1 -> Out1/1
  Pumping Station/15(L_11) -> [h1]
  Pumping Station/17(L_21) -> [h3]
  Pumping Station/18(L_22) -> [h4]
  Constant1/1 -> Switch4/1
  Constant2/1 -> Switch4/3
  [A] -> Switch4/2
  Switch4/1 -> Pumping Station/3(V_61)
  Pumping Station/16(L_12) -> [h2]
  Constant4/1 -> Switch5/3
  Constant3/1 -> Switch5/1
  [A] -> Switch5/2
  Switch5/1 -> Pumping Station/4(V_71)

== system inner_tanks_init/LU43 Pumping St. 1 ==
  note: Stop
  note: Stop
  note: Normal
  note: Stop
  note: Normal
  note: Normal
  In1 : Inport
  In2 : Inport  Port=2
  Constant{5,7..10} (5 alike) : Constant  Value=0
  Gain1 : Gain  Gain=100
  Gain2 : Gain  Gain=100
  Pumping Station : Subsystem
  Signal Specification1 : SignalSpecification  Unit=l/min
  Signal Specification2 : SignalSpecification  Unit=l/min
  Signal Specification3 : SignalSpecification  Unit=mm
  Signal Specification5 : SignalSpecification  Unit=mm
  Signal Specification6 : SignalSpecification  Commented=on  Unit=bar
  Switch1 : Switch  Criteria=u2 ~= 0
  Switch2 : Switch  Criteria=u2 ~= 0
  Switch3 : Switch  Criteria=u2 ~= 0
  Out2 : Outport  VectorParamsAs1DForOutWhenUnconnected=off
  Out5 : Outport  Port=2  VectorParamsAs1DForOutWhenUnconnected=off
  Out3 : Outport  Port=3  VectorParamsAs1DForOutWhenUnconnected=off
  Out4 : Outport  Port=4  VectorParamsAs1DForOutWhenUnconnected=off
  wires:
  Switch2/1 -> Pumping Station/7(Pu_3), Pumping Station/6(Pu_2), Pumping Station/5(Pu_1)
  [A] -> Switch1/2
  Constant7/1 -> Switch1/1
  Constant8/1 -> Switch1/3
  Switch3/1 -> Pumping Station/9(Pu_5), Pumping Station/8(Pu_4)
  Constant10/1 -> Switch3/1
  In1/1 -> Switch2/3
  [A] -> Switch2/2
  Constant9/1 -> Switch2/1
  In2/1 -> Switch3/3
  Gain2/1 -> Signal Specification3/1
  Constant5/1 -> Pumping Station/10(Pu_6)
  Signal Specification3/1 -> Out2/1
  [A] -> Switch3/2
  Pumping Station/5(dP2_ex) -> Gain2/1
  Switch1/1 -> Pumping Station/4(V_71), Pumping Station/3(V_61), Pumping Station/2(V_51), Pumping Station/1(V_31)
  Signal Specification1/1 -> Out3/1
  Signal Specification2/1 -> Out4/1
  Pumping Station/12(Q2_12) -> Signal Specification1/1
  Pumping Station/13(Q2_51) -> Signal Specification2/1
  Pumping Station/6(dP2_in) -> Gain1/1
  Signal Specification5/1 -> Out5/1
  Gain1/1 -> Signal Specification5/1

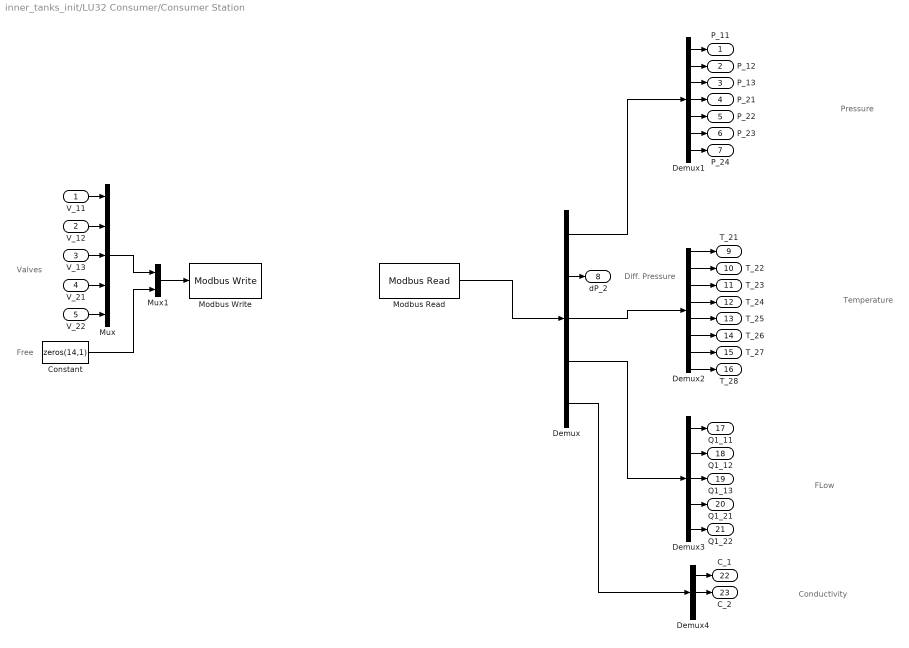
== system inner_tanks_init/LU32 Consumer/Consumer Station ==
  note: Pressure
  note: Temperature
  note: FLow
  note: Conductivity
  note: Valves
  note: Diff. Pressure
  note: Free
  V_11 : Inport
  V_12 : Inport  Port=2
  V_13 : Inport  Port=3
  V_21 : Inport  Port=4
  V_22 : Inport  Port=5
  Constant : Constant  Value=zeros(14,1)
  Demux : Demux  Outputs=[7 1 8 5 3]
  Demux1 : Demux  Outputs=7
  Demux2 : Demux  Outputs=8
  Demux3 : Demux  Outputs=5
  Demux4 : Demux  Outputs=3
  Modbus Read : modbusMatLib/Modbus Read  registry=0  ipAddress='192.168.100.32'  port=502
  Modbus Write : modbusMatLib/Modbus Write  registry=001  port=502  ipAddress='192.168.100.32'
  Mux : Mux  Inputs=5
  Mux1 : Mux  Inputs=2
  P_11 : Outport  VectorParamsAs1DForOutWhenUnconnected=off
  P_12 : Outport  Port=2  VectorParamsAs1DForOutWhenUnconnected=off
  P_13 : Outport  Port=3  VectorParamsAs1DForOutWhenUnconnected=off
  P_21 : Outport  Port=4  VectorParamsAs1DForOutWhenUnconnected=off
  P_22 : Outport  Port=5  VectorParamsAs1DForOutWhenUnconnected=off
  P_23 : Outport  Port=6  VectorParamsAs1DForOutWhenUnconnected=off
  P_24 : Outport  Port=7  VectorParamsAs1DForOutWhenUnconnected=off
  dP_2 : Outport  Port=8  VectorParamsAs1DForOutWhenUnconnected=off
  T_21 : Outport  Port=9  VectorParamsAs1DForOutWhenUnconnected=off
  T_22 : Outport  Port=10  VectorParamsAs1DForOutWhenUnconnected=off
  T_23 : Outport  Port=11  VectorParamsAs1DForOutWhenUnconnected=off
  T_24 : Outport  Port=12  VectorParamsAs1DForOutWhenUnconnected=off
  T_25 : Outport  Port=13  VectorParamsAs1DForOutWhenUnconnected=off
  T_26 : Outport  Port=14  VectorParamsAs1DForOutWhenUnconnected=off
  T_27 : Outport  Port=15  VectorParamsAs1DForOutWhenUnconnected=off
  T_28 : Outport  Port=16  VectorParamsAs1DForOutWhenUnconnected=off
  Q1_11 : Outport  Port=17  VectorParamsAs1DForOutWhenUnconnected=off
  Q1_12 : Outport  Port=18  VectorParamsAs1DForOutWhenUnconnected=off
  Q1_13 : Outport  Port=19  VectorParamsAs1DForOutWhenUnconnected=off
  Q1_21 : Outport  Port=20  VectorParamsAs1DForOutWhenUnconnected=off
  Q1_22 : Outport  Port=21  VectorParamsAs1DForOutWhenUnconnected=off
  C_1 : Outport  Port=22  VectorParamsAs1DForOutWhenUnconnected=off
  C_2 : Outport  Port=23  VectorParamsAs1DForOutWhenUnconnected=off
  wires:
  Mux/1 -> Mux1/1
  Mux1/1 -> Modbus Write/1
  Constant/1 -> Mux1/2
  Demux1/5 -> P_22/1
  V_12/1 -> Mux/2
  Demux1/6 -> P_23/1
  Demux1/3 -> P_13/1
  Demux1/4 -> P_21/1
  V_13/1 -> Mux/3
  Demux3/2 -> Q1_12/1
  Demux3/5 -> Q1_22/1
  Demux/2 -> dP_2/1
  Demux3/1 -> Q1_11/1
  Demux1/2 -> P_12/1
  Demux2/5 -> T_25/1
  Demux4/1 -> C_1/1
  V_21/1 -> Mux/4
  Demux3/3 -> Q1_13/1
  Demux1/1 -> P_11/1
  Demux3/4 -> Q1_21/1
  V_11/1 -> Mux/1
  Demux2/4 -> T_24/1
  Demux2/3 -> T_23/1
  Demux2/2 -> T_22/1
  Demux2/1 -> T_21/1
  Demux1/7 -> P_24/1
  V_22/1 -> Mux/5
  Demux2/7 -> T_27/1
  Demux/5 -> Demux4/1
  Demux/1 -> Demux1/1
  Demux2/8 -> T_28/1
  Demux4/2 -> C_2/1
  Demux/3 -> Demux2/1
  Demux/4 -> Demux3/1
  Modbus Read/1 -> Demux/1
  Demux2/6 -> T_26/1

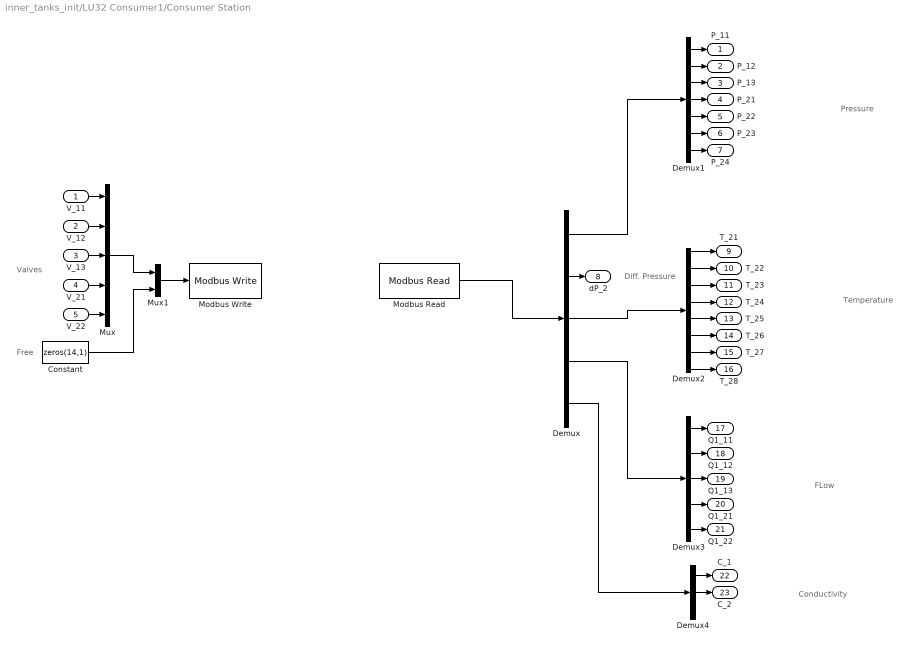
== system inner_tanks_init/LU32 Consumer1/Consumer Station ==
  note: Pressure
  note: Temperature
  note: FLow
  note: Conductivity
  note: Valves
  note: Diff. Pressure
  note: Free
  V_11 : Inport
  V_12 : Inport  Port=2
  V_13 : Inport  Port=3
  V_21 : Inport  Port=4
  V_22 : Inport  Port=5
  Constant : Constant  Value=zeros(14,1)
  Demux : Demux  Outputs=[7 1 8 5 3]
  Demux1 : Demux  Outputs=7
  Demux2 : Demux  Outputs=8
  Demux3 : Demux  Outputs=5
  Demux4 : Demux  Outputs=3
  Modbus Read : modbusMatLib/Modbus Read  registry=0  ipAddress='192.168.100.33'  port=502
  Modbus Write : modbusMatLib/Modbus Write  registry=001  port=502  ipAddress='192.168.100.33'
  Mux : Mux  Inputs=5
  Mux1 : Mux  Inputs=2
  P_11 : Outport  VectorParamsAs1DForOutWhenUnconnected=off
  P_12 : Outport  Port=2  VectorParamsAs1DForOutWhenUnconnected=off
  P_13 : Outport  Port=3  VectorParamsAs1DForOutWhenUnconnected=off
  P_21 : Outport  Port=4  VectorParamsAs1DForOutWhenUnconnected=off
  P_22 : Outport  Port=5  VectorParamsAs1DForOutWhenUnconnected=off
  P_23 : Outport  Port=6  VectorParamsAs1DForOutWhenUnconnected=off
  P_24 : Outport  Port=7  VectorParamsAs1DForOutWhenUnconnected=off
  dP_2 : Outport  Port=8  VectorParamsAs1DForOutWhenUnconnected=off
  T_21 : Outport  Port=9  VectorParamsAs1DForOutWhenUnconnected=off
  T_22 : Outport  Port=10  VectorParamsAs1DForOutWhenUnconnected=off
  T_23 : Outport  Port=11  VectorParamsAs1DForOutWhenUnconnected=off
  T_24 : Outport  Port=12  VectorParamsAs1DForOutWhenUnconnected=off
  T_25 : Outport  Port=13  VectorParamsAs1DForOutWhenUnconnected=off
  T_26 : Outport  Port=14  VectorParamsAs1DForOutWhenUnconnected=off
  T_27 : Outport  Port=15  VectorParamsAs1DForOutWhenUnconnected=off
  T_28 : Outport  Port=16  VectorParamsAs1DForOutWhenUnconnected=off
  Q1_11 : Outport  Port=17  VectorParamsAs1DForOutWhenUnconnected=off
  Q1_12 : Outport  Port=18  VectorParamsAs1DForOutWhenUnconnected=off
  Q1_13 : Outport  Port=19  VectorParamsAs1DForOutWhenUnconnected=off
  Q1_21 : Outport  Port=20  VectorParamsAs1DForOutWhenUnconnected=off
  Q1_22 : Outport  Port=21  VectorParamsAs1DForOutWhenUnconnected=off
  C_1 : Outport  Port=22  VectorParamsAs1DForOutWhenUnconnected=off
  C_2 : Outport  Port=23  VectorParamsAs1DForOutWhenUnconnected=off
  wires:
  Mux/1 -> Mux1/1
  Mux1/1 -> Modbus Write/1
  Constant/1 -> Mux1/2
  Demux1/5 -> P_22/1
  V_12/1 -> Mux/2
  Demux1/6 -> P_23/1
  Demux1/3 -> P_13/1
  Demux1/4 -> P_21/1
  V_13/1 -> Mux/3
  Demux3/2 -> Q1_12/1
  Demux3/5 -> Q1_22/1
  Demux/2 -> dP_2/1
  Demux3/1 -> Q1_11/1
  Demux1/2 -> P_12/1
  Demux2/5 -> T_25/1
  Demux4/1 -> C_1/1
  V_21/1 -> Mux/4
  Demux3/3 -> Q1_13/1
  Demux1/1 -> P_11/1
  Demux3/4 -> Q1_21/1
  V_11/1 -> Mux/1
  Demux2/4 -> T_24/1
  Demux2/3 -> T_23/1
  Demux2/2 -> T_22/1
  Demux2/1 -> T_21/1
  Demux1/7 -> P_24/1
  V_22/1 -> Mux/5
  Demux2/7 -> T_27/1
  Demux/5 -> Demux4/1
  Demux/1 -> Demux1/1
  Demux2/8 -> T_28/1
  Demux4/2 -> C_2/1
  Demux/3 -> Demux2/1
  Demux/4 -> Demux3/1
  Modbus Read/1 -> Demux/1
  Demux2/6 -> T_26/1

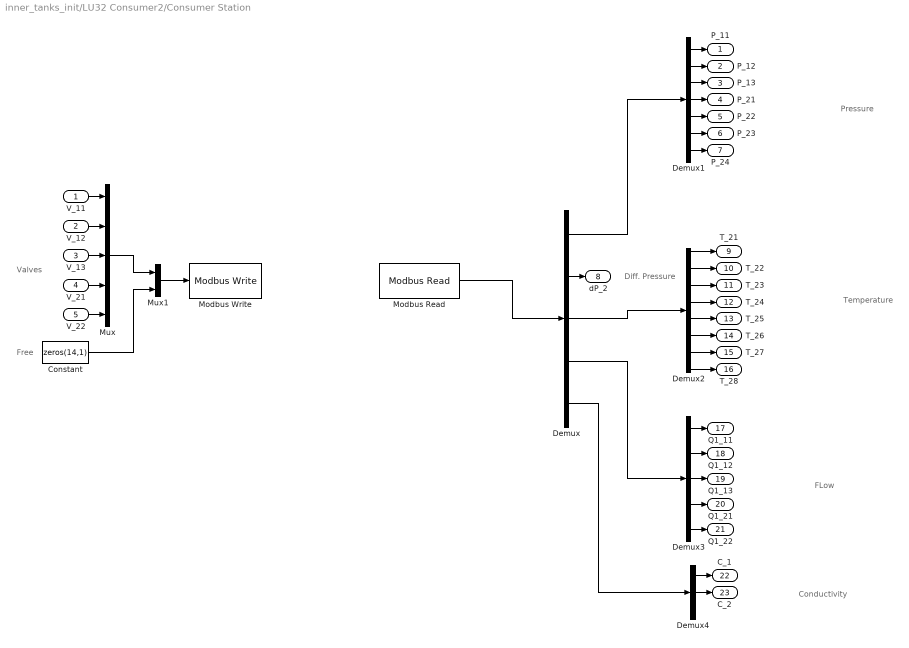
== system inner_tanks_init/LU32 Consumer2/Consumer Station ==
  note: Pressure
  note: Temperature
  note: FLow
  note: Conductivity
  note: Valves
  note: Diff. Pressure
  note: Free
  V_11 : Inport
  V_12 : Inport  Port=2
  V_13 : Inport  Port=3
  V_21 : Inport  Port=4
  V_22 : Inport  Port=5
  Constant : Constant  Value=zeros(14,1)
  Demux : Demux  Outputs=[7 1 8 5 3]
  Demux1 : Demux  Outputs=7
  Demux2 : Demux  Outputs=8
  Demux3 : Demux  Outputs=5
  Demux4 : Demux  Outputs=3
  Modbus Read : modbusMatLib/Modbus Read  registry=0  ipAddress='192.168.100.32'  port=502
  Modbus Write : modbusMatLib/Modbus Write  registry=001  port=502  ipAddress='192.168.100.32'
  Mux : Mux  Inputs=5
  Mux1 : Mux  Inputs=2
  P_11 : Outport  VectorParamsAs1DForOutWhenUnconnected=off
  P_12 : Outport  Port=2  VectorParamsAs1DForOutWhenUnconnected=off
  P_13 : Outport  Port=3  VectorParamsAs1DForOutWhenUnconnected=off
  P_21 : Outport  Port=4  VectorParamsAs1DForOutWhenUnconnected=off
  P_22 : Outport  Port=5  VectorParamsAs1DForOutWhenUnconnected=off
  P_23 : Outport  Port=6  VectorParamsAs1DForOutWhenUnconnected=off
  P_24 : Outport  Port=7  VectorParamsAs1DForOutWhenUnconnected=off
  dP_2 : Outport  Port=8  VectorParamsAs1DForOutWhenUnconnected=off
  T_21 : Outport  Port=9  VectorParamsAs1DForOutWhenUnconnected=off
  T_22 : Outport  Port=10  VectorParamsAs1DForOutWhenUnconnected=off
  T_23 : Outport  Port=11  VectorParamsAs1DForOutWhenUnconnected=off
  T_24 : Outport  Port=12  VectorParamsAs1DForOutWhenUnconnected=off
  T_25 : Outport  Port=13  VectorParamsAs1DForOutWhenUnconnected=off
  T_26 : Outport  Port=14  VectorParamsAs1DForOutWhenUnconnected=off
  T_27 : Outport  Port=15  VectorParamsAs1DForOutWhenUnconnected=off
  T_28 : Outport  Port=16  VectorParamsAs1DForOutWhenUnconnected=off
  Q1_11 : Outport  Port=17  VectorParamsAs1DForOutWhenUnconnected=off
  Q1_12 : Outport  Port=18  VectorParamsAs1DForOutWhenUnconnected=off
  Q1_13 : Outport  Port=19  VectorParamsAs1DForOutWhenUnconnected=off
  Q1_21 : Outport  Port=20  VectorParamsAs1DForOutWhenUnconnected=off
  Q1_22 : Outport  Port=21  VectorParamsAs1DForOutWhenUnconnected=off
  C_1 : Outport  Port=22  VectorParamsAs1DForOutWhenUnconnected=off
  C_2 : Outport  Port=23  VectorParamsAs1DForOutWhenUnconnected=off
  wires:
  Mux/1 -> Mux1/1
  Mux1/1 -> Modbus Write/1
  Constant/1 -> Mux1/2
  Demux1/5 -> P_22/1
  V_12/1 -> Mux/2
  Demux1/6 -> P_23/1
  Demux1/3 -> P_13/1
  Demux1/4 -> P_21/1
  V_13/1 -> Mux/3
  Demux3/2 -> Q1_12/1
  Demux3/5 -> Q1_22/1
  Demux/2 -> dP_2/1
  Demux3/1 -> Q1_11/1
  Demux1/2 -> P_12/1
  Demux2/5 -> T_25/1
  Demux4/1 -> C_1/1
  V_21/1 -> Mux/4
  Demux3/3 -> Q1_13/1
  Demux1/1 -> P_11/1
  Demux3/4 -> Q1_21/1
  V_11/1 -> Mux/1
  Demux2/4 -> T_24/1
  Demux2/3 -> T_23/1
  Demux2/2 -> T_22/1
  Demux2/1 -> T_21/1
  Demux1/7 -> P_24/1
  V_22/1 -> Mux/5
  Demux2/7 -> T_27/1
  Demux/5 -> Demux4/1
  Demux/1 -> Demux1/1
  Demux2/8 -> T_28/1
  Demux4/2 -> C_2/1
  Demux/3 -> Demux2/1
  Demux/4 -> Demux3/1
  Modbus Read/1 -> Demux/1
  Demux2/6 -> T_26/1

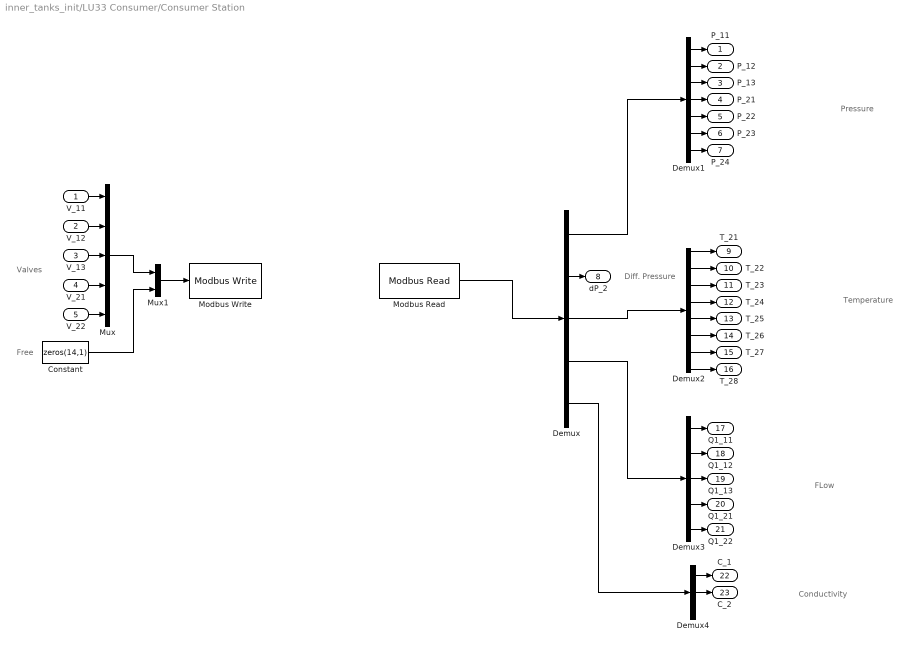
== system inner_tanks_init/LU33 Consumer/Consumer Station ==
  note: Pressure
  note: Temperature
  note: FLow
  note: Conductivity
  note: Valves
  note: Diff. Pressure
  note: Free
  V_11 : Inport
  V_12 : Inport  Port=2
  V_13 : Inport  Port=3
  V_21 : Inport  Port=4
  V_22 : Inport  Port=5
  Constant : Constant  Value=zeros(14,1)
  Demux : Demux  Outputs=[7 1 8 5 3]
  Demux1 : Demux  Outputs=7
  Demux2 : Demux  Outputs=8
  Demux3 : Demux  Outputs=5
  Demux4 : Demux  Outputs=3
  Modbus Read : modbusMatLib/Modbus Read  registry=0  ipAddress='192.168.100.33'  port=502
  Modbus Write : modbusMatLib/Modbus Write  registry=001  port=502  ipAddress='192.168.100.33'
  Mux : Mux  Inputs=5
  Mux1 : Mux  Inputs=2
  P_11 : Outport  VectorParamsAs1DForOutWhenUnconnected=off
  P_12 : Outport  Port=2  VectorParamsAs1DForOutWhenUnconnected=off
  P_13 : Outport  Port=3  VectorParamsAs1DForOutWhenUnconnected=off
  P_21 : Outport  Port=4  VectorParamsAs1DForOutWhenUnconnected=off
  P_22 : Outport  Port=5  VectorParamsAs1DForOutWhenUnconnected=off
  P_23 : Outport  Port=6  VectorParamsAs1DForOutWhenUnconnected=off
  P_24 : Outport  Port=7  VectorParamsAs1DForOutWhenUnconnected=off
  dP_2 : Outport  Port=8  VectorParamsAs1DForOutWhenUnconnected=off
  T_21 : Outport  Port=9  VectorParamsAs1DForOutWhenUnconnected=off
  T_22 : Outport  Port=10  VectorParamsAs1DForOutWhenUnconnected=off
  T_23 : Outport  Port=11  VectorParamsAs1DForOutWhenUnconnected=off
  T_24 : Outport  Port=12  VectorParamsAs1DForOutWhenUnconnected=off
  T_25 : Outport  Port=13  VectorParamsAs1DForOutWhenUnconnected=off
  T_26 : Outport  Port=14  VectorParamsAs1DForOutWhenUnconnected=off
  T_27 : Outport  Port=15  VectorParamsAs1DForOutWhenUnconnected=off
  T_28 : Outport  Port=16  VectorParamsAs1DForOutWhenUnconnected=off
  Q1_11 : Outport  Port=17  VectorParamsAs1DForOutWhenUnconnected=off
  Q1_12 : Outport  Port=18  VectorParamsAs1DForOutWhenUnconnected=off
  Q1_13 : Outport  Port=19  VectorParamsAs1DForOutWhenUnconnected=off
  Q1_21 : Outport  Port=20  VectorParamsAs1DForOutWhenUnconnected=off
  Q1_22 : Outport  Port=21  VectorParamsAs1DForOutWhenUnconnected=off
  C_1 : Outport  Port=22  VectorParamsAs1DForOutWhenUnconnected=off
  C_2 : Outport  Port=23  VectorParamsAs1DForOutWhenUnconnected=off
  wires:
  Mux/1 -> Mux1/1
  Mux1/1 -> Modbus Write/1
  Constant/1 -> Mux1/2
  Demux1/5 -> P_22/1
  V_12/1 -> Mux/2
  Demux1/6 -> P_23/1
  Demux1/3 -> P_13/1
  Demux1/4 -> P_21/1
  V_13/1 -> Mux/3
  Demux3/2 -> Q1_12/1
  Demux3/5 -> Q1_22/1
  Demux/2 -> dP_2/1
  Demux3/1 -> Q1_11/1
  Demux1/2 -> P_12/1
  Demux2/5 -> T_25/1
  Demux4/1 -> C_1/1
  V_21/1 -> Mux/4
  Demux3/3 -> Q1_13/1
  Demux1/1 -> P_11/1
  Demux3/4 -> Q1_21/1
  V_11/1 -> Mux/1
  Demux2/4 -> T_24/1
  Demux2/3 -> T_23/1
  Demux2/2 -> T_22/1
  Demux2/1 -> T_21/1
  Demux1/7 -> P_24/1
  V_22/1 -> Mux/5
  Demux2/7 -> T_27/1
  Demux/5 -> Demux4/1
  Demux/1 -> Demux1/1
  Demux2/8 -> T_28/1
  Demux4/2 -> C_2/1
  Demux/3 -> Demux2/1
  Demux/4 -> Demux3/1
  Modbus Read/1 -> Demux/1
  Demux2/6 -> T_26/1

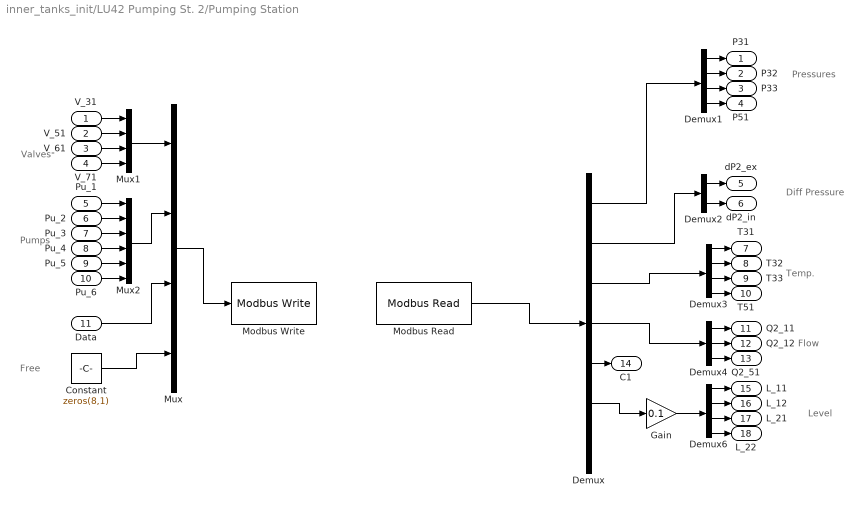
== system inner_tanks_init/LU42 Pumping St. 2/Pumping Station ==
  note: Free
  note: Pumps
  note: Valves
  note: Flow
  note: Temp.
  note: Diff Pressure
  note: Pressures
  note: Level
  V_31 : Inport
  V_51 : Inport  Port=2
  V_61 : Inport  Port=3
  V_71 : Inport  Port=4
  Pu_1 : Inport  Port=5
  Pu_2 : Inport  Port=6
  Pu_3 : Inport  Port=7
  Pu_4 : Inport  Port=8
  Pu_5 : Inport  Port=9
  Pu_6 : Inport  Port=10
  Data : Inport  Port=11
  Constant : Constant  Value=zeros(8,1)
  Demux : Demux  Outputs=[4 2 4 3 1 4 6]
  Demux1 : Demux
  Demux2 : Demux  Outputs=2
  Demux3 : Demux
  Demux4 : Demux  Outputs=3
  Demux6 : Demux
  Gain : Gain  Gain=0.1
  Modbus Read : modbusMatLib/Modbus Read  registry=0  ipAddress='192.168.100.42'  port=502
  Modbus Write : modbusMatLib/Modbus Write  registry=001  port=502  ipAddress='192.168.100.42'
  Mux : Mux
  Mux1 : Mux
  Mux2 : Mux  Inputs=6
  P31 : Outport  VectorParamsAs1DForOutWhenUnconnected=off
  P32 : Outport  Port=2  VectorParamsAs1DForOutWhenUnconnected=off
  P33 : Outport  Port=3  VectorParamsAs1DForOutWhenUnconnected=off
  P51 : Outport  Port=4  VectorParamsAs1DForOutWhenUnconnected=off
  dP2_ex : Outport  Port=5  VectorParamsAs1DForOutWhenUnconnected=off
  dP2_in : Outport  Port=6  VectorParamsAs1DForOutWhenUnconnected=off
  T31 : Outport  Port=7  VectorParamsAs1DForOutWhenUnconnected=off
  T32 : Outport  Port=8  VectorParamsAs1DForOutWhenUnconnected=off
  T33 : Outport  Port=9  VectorParamsAs1DForOutWhenUnconnected=off
  T51 : Outport  Port=10  VectorParamsAs1DForOutWhenUnconnected=off
  Q2_11 : Outport  Port=11  VectorParamsAs1DForOutWhenUnconnected=off
  Q2_12 : Outport  Port=12  VectorParamsAs1DForOutWhenUnconnected=off
  Q2_51 : Outport  Port=13  VectorParamsAs1DForOutWhenUnconnected=off
  C1 : Outport  Port=14  VectorParamsAs1DForOutWhenUnconnected=off
  L_11 : Outport  Port=15  VectorParamsAs1DForOutWhenUnconnected=off
  L_12 : Outport  Port=16  VectorParamsAs1DForOutWhenUnconnected=off
  L_21 : Outport  Port=17  VectorParamsAs1DForOutWhenUnconnected=off
  L_22 : Outport  Port=18  VectorParamsAs1DForOutWhenUnconnected=off
  wires:
  Demux4/1 -> Q2_11/1
  Demux/2 -> Demux2/1
  Demux/4 -> Demux4/1
  Demux2/1 -> dP2_ex/1
  Demux/3 -> Demux3/1
  Demux/1 -> Demux1/1
  Demux3/4 -> T51/1
  Demux1/4 -> P51/1
  Demux3/2 -> T32/1
  Modbus Read/1 -> Demux/1
  Demux6/1 -> L_11/1
  Demux6/2 -> L_12/1
  Demux4/3 -> Q2_51/1
  Demux4/2 -> Q2_12/1
  Demux6/3 -> L_21/1
  Demux6/4 -> L_22/1
  Demux3/3 -> T33/1
  Demux1/1 -> P31/1
  Demux1/2 -> P32/1
  Demux/5 -> C1/1
  Demux1/3 -> P33/1
  Demux2/2 -> dP2_in/1
  Demux3/1 -> T31/1
  Mux/1 -> Modbus Write/1
  Mux1/1 -> Mux/1
  V_31/1 -> Mux1/1
  V_51/1 -> Mux1/2
  V_61/1 -> Mux1/3
  V_71/1 -> Mux1/4
  Pu_4/1 -> Mux2/4
  Pu_3/1 -> Mux2/3
  Pu_1/1 -> Mux2/1
  Pu_2/1 -> Mux2/2
  Mux2/1 -> Mux/2
  Pu_5/1 -> Mux2/5
  Pu_6/1 -> Mux2/6
  Data/1 -> Mux/3
  Constant/1 -> Mux/4
  Gain/1 -> Demux6/1
  Demux/6 -> Gain/1

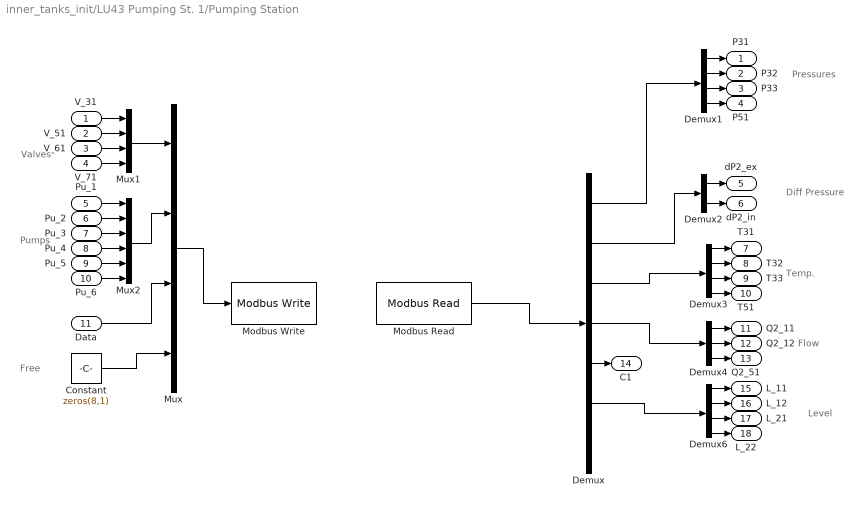
== system inner_tanks_init/LU43 Pumping St. 1/Pumping Station ==
  note: Free
  note: Pumps
  note: Valves
  note: Flow
  note: Temp.
  note: Diff Pressure
  note: Pressures
  note: Level
  V_31 : Inport
  V_51 : Inport  Port=2
  V_61 : Inport  Port=3
  V_71 : Inport  Port=4
  Pu_1 : Inport  Port=5
  Pu_2 : Inport  Port=6
  Pu_3 : Inport  Port=7
  Pu_4 : Inport  Port=8
  Pu_5 : Inport  Port=9
  Pu_6 : Inport  Port=10
  Data : Inport  Port=11
  Constant : Constant  Value=zeros(8,1)
  Demux : Demux  Outputs=[4 2 4 3 1 4 6]
  Demux1 : Demux
  Demux2 : Demux  Outputs=2
  Demux3 : Demux
  Demux4 : Demux  Outputs=3
  Demux6 : Demux
  Modbus Read : modbusMatLib/Modbus Read  registry=0  ipAddress='192.168.100.43'  port=502
  Modbus Write : modbusMatLib/Modbus Write  registry=001  port=502  ipAddress='192.168.100.43'
  Mux : Mux
  Mux1 : Mux
  Mux2 : Mux  Inputs=6
  P31 : Outport  VectorParamsAs1DForOutWhenUnconnected=off
  P32 : Outport  Port=2  VectorParamsAs1DForOutWhenUnconnected=off
  P33 : Outport  Port=3  VectorParamsAs1DForOutWhenUnconnected=off
  P51 : Outport  Port=4  VectorParamsAs1DForOutWhenUnconnected=off
  dP2_ex : Outport  Port=5  VectorParamsAs1DForOutWhenUnconnected=off
  dP2_in : Outport  Port=6  VectorParamsAs1DForOutWhenUnconnected=off
  T31 : Outport  Port=7  VectorParamsAs1DForOutWhenUnconnected=off
  T32 : Outport  Port=8  VectorParamsAs1DForOutWhenUnconnected=off
  T33 : Outport  Port=9  VectorParamsAs1DForOutWhenUnconnected=off
  T51 : Outport  Port=10  VectorParamsAs1DForOutWhenUnconnected=off
  Q2_11 : Outport  Port=11  VectorParamsAs1DForOutWhenUnconnected=off
  Q2_12 : Outport  Port=12  VectorParamsAs1DForOutWhenUnconnected=off
  Q2_51 : Outport  Port=13  VectorParamsAs1DForOutWhenUnconnected=off
  C1 : Outport  Port=14  VectorParamsAs1DForOutWhenUnconnected=off
  L_11 : Outport  Port=15  VectorParamsAs1DForOutWhenUnconnected=off
  L_12 : Outport  Port=16  VectorParamsAs1DForOutWhenUnconnected=off
  L_21 : Outport  Port=17  VectorParamsAs1DForOutWhenUnconnected=off
  L_22 : Outport  Port=18  VectorParamsAs1DForOutWhenUnconnected=off
  wires:
  Demux4/1 -> Q2_11/1
  Demux/2 -> Demux2/1
  Demux/4 -> Demux4/1
  Demux2/1 -> dP2_ex/1
  Demux/3 -> Demux3/1
  Demux/6 -> Demux6/1
  Demux/1 -> Demux1/1
  Demux3/4 -> T51/1
  Demux1/4 -> P51/1
  Demux3/2 -> T32/1
  Modbus Read/1 -> Demux/1
  Demux6/1 -> L_11/1
  Demux6/2 -> L_12/1
  Demux4/3 -> Q2_51/1
  Demux4/2 -> Q2_12/1
  Demux6/3 -> L_21/1
  Demux6/4 -> L_22/1
  Demux3/3 -> T33/1
  Demux1/1 -> P31/1
  Demux1/2 -> P32/1
  Demux/5 -> C1/1
  Demux1/3 -> P33/1
  Demux2/2 -> dP2_in/1
  Demux3/1 -> T31/1
  Mux/1 -> Modbus Write/1
  Mux1/1 -> Mux/1
  V_31/1 -> Mux1/1
  V_51/1 -> Mux1/2
  V_61/1 -> Mux1/3
  V_71/1 -> Mux1/4
  Pu_4/1 -> Mux2/4
  Pu_3/1 -> Mux2/3
  Pu_1/1 -> Mux2/1
  Pu_2/1 -> Mux2/2
  Mux2/1 -> Mux/2
  Pu_5/1 -> Mux2/5
  Pu_6/1 -> Mux2/6
  Data/1 -> Mux/3
  Constant/1 -> Mux/4

== matlab function inner_tanks_init/MATLAB Function2 ==
  data: dp_tank1 input; pump_aux_setting output; old_setting input
function pump_aux_setting = controller(dp_tank1,old_setting)

    if dp_tank1<300                       
        pump_aux_setting = 8;                               
    elseif  dp_tank1 > 550
        pump_aux_setting = 0;
    else
        pump_aux_setting = old_setting;
    end
end
